simulink model "rocket_model"  (R2024a)
settings: Solver=VariableStepAuto  StartTime=0.0  StopTime=3  FixedStep=sample_time  RelTol=1e-3
undefined symbols (not defined in the file): armTVC, c_d, contact, fractalcoef, g, m, max_angle, sample_time
libraries: sharedtransform x4, sharedutil x3, slpidlib x2, aerolibutil x2, shared6dof x1, simulink x1, mspsensorlib x1, uavutilslib x1
settings Model: Creator=tommy  LastModifiedBy=tommy

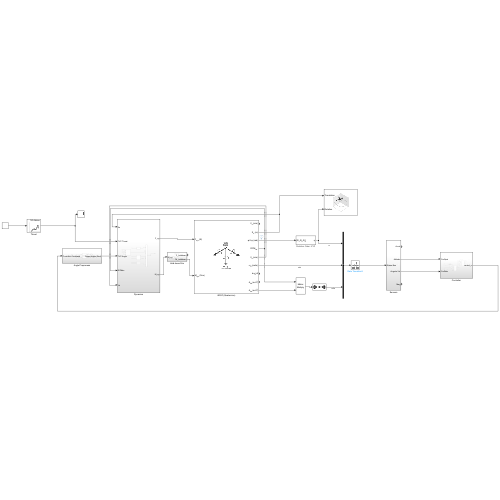
[thumbnail: Simulink's stored preview of the top-level diagram]
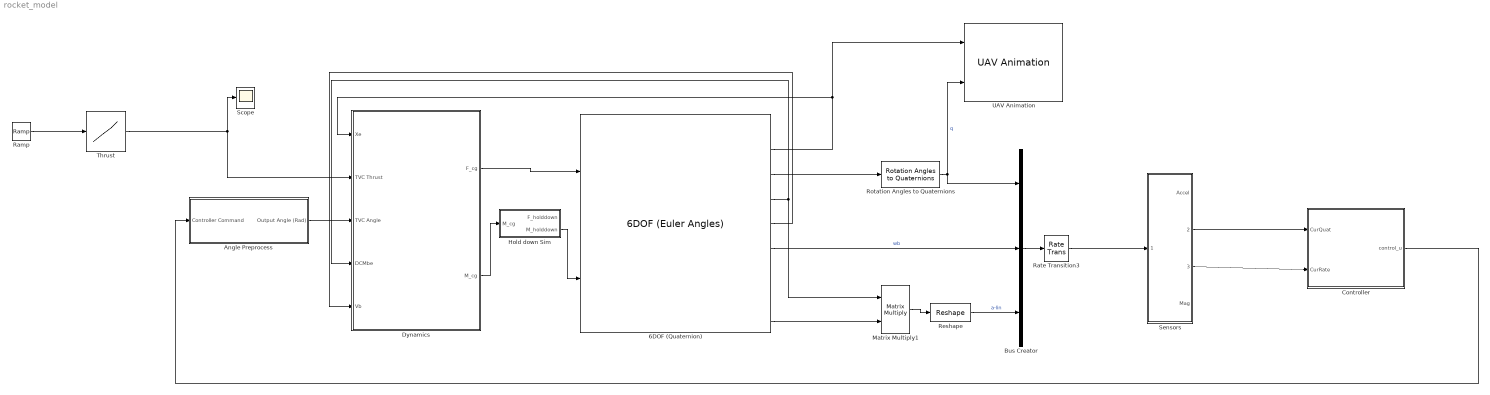
== system rocket_model ==
  6DOF (Quaternion) : shared6dof/6DOF (Euler Angles)  units=Metric (MKS)  mtype=Fixed  rep=Quaternion  xme_0=[0 0 0]  Vm_0=[0 0 0]  eul_0=[0, 0.2, 0]  pm_0=[0 0 0]  mass_0=m  mass_e=0.5  mass_f=2.0  inertia=inertia  inertia_e=eye(3)  inertia_f=2*eye(3)  k_quat=1  vre_flag=on  abi_flag=on  aMode=0  xme_statename=''  Vm_statename=''  eul_statename=''  quat_statename=''  pm_statename=''  mass_statename=''
      settings: LibrarySourceBlock=aerolib6dof2/6DOF (Quaternion)
  Angle Preprocess : Subsystem
  Bus Creator : BusCreator  Inputs=3
  Controller : Subsystem
  Dynamics : Subsystem
  Hold down Sim : Subsystem
  Matrix Multiply1 : Product  Multiplication=Matrix(*)
  Ramp : simulink/Sources/Ramp  slope=1  start=0  InitialOutput=0
  Rate Transition3 : RateTransition  OutPortSampleTime=sample_time
  Reshape : Reshape  OutputDimensionality=Row vector (2-D)
  Rotation Angles to Quaternions : sharedtransform/Rotation Angles to Quaternions  rotationOrder=XYZ  aMode=aMode
  Scope : Scope
  Sensors : Subsystem
  Thrust : Lookup_n-D  NumberOfTableDimensions=1  BreakpointsForDimension1=[0;0.15;0.186;0.206;0.242;0.252;0.277;0.333;0.359;0.374;0.394;0.435;0.476;0.521;0.643;0.725;0.821;0.898;1.025;1.142;1.259;1.396;1.569;1.757;1.895;2.027;2.042;2.052;2.063;2.09;4;10]  Table=[0;1.371;1.92;3.387;5.587;7.422;8.705;13.474;15.858;16.592;18.609;21.544;24.661;26.44;21.72;20.432;19.511;18.958;18.219;18.032;17.844;17.472;17.282;17.275;17.086;17.816;12.494;8.457;4.97;0;0;0]  InterpMethod=Akima spline  InternalRulePriority=Speed  RndMeth=Simplest
  UAV Animation : uavutilslib/UAV Animation  UAVType=Multirotor  UAVSize=1  InertialZDirection=Down  SampleTime=-1
  wires:
  Thrust/1 -> Dynamics/2(TVC Thrust), Scope/1
  6DOF (Quaternion)/4 -> Dynamics/4(DCMbe), Matrix Multiply1/1
  6DOF (Quaternion)/5 -> Dynamics/5(Vb)
  Ramp/1 -> Thrust/1
  6DOF (Quaternion)/2 -> UAV Animation/1, Dynamics/1(Xe)
  6DOF (Quaternion)/3 -> Rotation Angles to Quaternions/1
  Angle Preprocess/1(Output Angle (Rad)) -> Dynamics/3(TVC Angle)
  Controller/1(control_u) -> Angle Preprocess/1(Controller Command)
  Dynamics/2(M_cg) -> Hold down Sim/1(M_cg)
  Hold down Sim/2(M_holddown) -> 6DOF (Quaternion)/2
  6DOF (Quaternion)/9 -> Matrix Multiply1/2
  Matrix Multiply1/1 -> Reshape/1
  Dynamics/1(F_cg) -> 6DOF (Quaternion)/1
  Rotation Angles to Quaternions/1 -> Bus Creator/1, UAV Animation/2  "q"
  Reshape/1 -> Bus Creator/3  "a-lin"
  6DOF (Quaternion)/6 -> Bus Creator/2  "wb"
  Bus Creator/1 -> Rate Transition3/1
  Sensors/2(Attitude) -> Controller/1(CurQuat)
  Sensors/3(Angular Vel) -> Controller/2(CurRate)
  Rate Transition3/1 -> Sensors/1(States Bus)

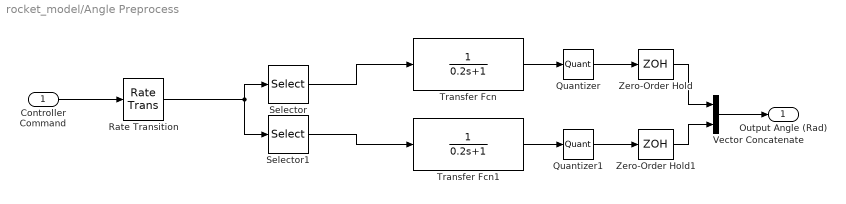
== system rocket_model/Angle Preprocess ==
  Controller Command : Inport
  Quantizer : Quantizer  QuantizationInterval=0.01745329251
  Quantizer1 : Quantizer  QuantizationInterval=0.01745329251
  Rate Transition : RateTransition  OutPortSampleTime=1/100
  Selector : Selector  InputPortWidth=3  IndexOptions=Index vector (dialog)  Indices=[1]  OutputSizes=1
  Selector1 : Selector  InputPortWidth=3  IndexOptions=Index vector (dialog)  Indices=[2]  OutputSizes=1
  Transfer Fcn : TransferFcn  Denominator=[0.2 1]
  Transfer Fcn1 : TransferFcn  Denominator=[0.2 1]
  Vector Concatenate : Concatenate
  Zero-Order Hold : ZeroOrderHold  SampleTime=1/100
  Zero-Order Hold1 : ZeroOrderHold  SampleTime=1/100
  Output Angle (Rad) : Outport
  wires:
  Vector Concatenate/1 -> Output Angle (Rad)/1
  Controller Command/1 -> Rate Transition/1
  Selector1/1 -> Transfer Fcn1/1
  Transfer Fcn/1 -> Quantizer/1
  Selector/1 -> Transfer Fcn/1
  Rate Transition/1 -> Selector1/1, Selector/1
  Quantizer/1 -> Zero-Order Hold/1
  Zero-Order Hold/1 -> Vector Concatenate/1
  Quantizer1/1 -> Zero-Order Hold1/1
  Zero-Order Hold1/1 -> Vector Concatenate/2
  Transfer Fcn1/1 -> Quantizer1/1

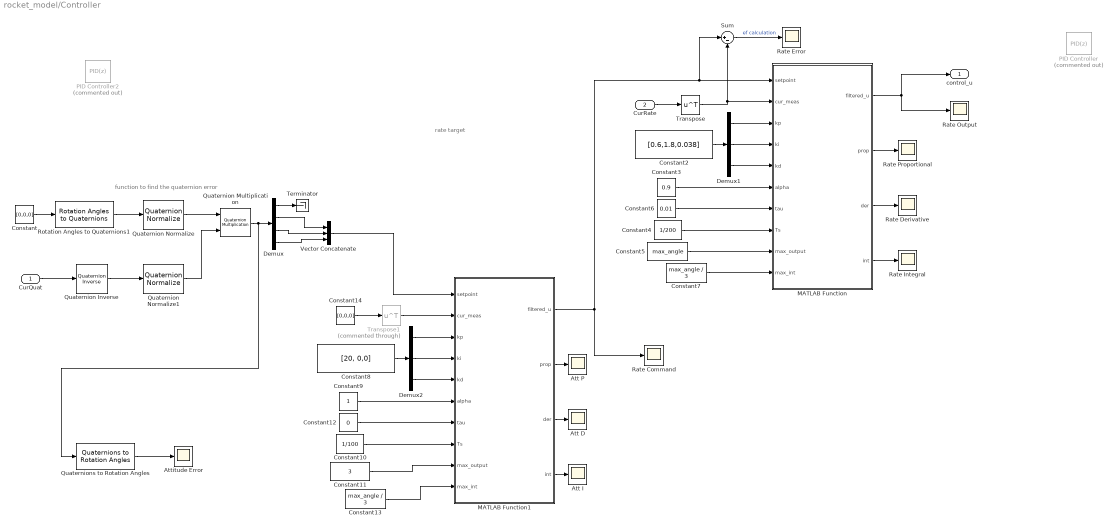
== system rocket_model/Controller ==
  note: rate target
  note: function to find the quaternion error
  CurQuat : Inport
  CurRate : Inport  Port=2
  Att D : Scope
  Att I : Scope
  Att P : Scope
  Attitude Error : Scope
  Constant : Constant  Value=[0,0,0]
  Constant10 : Constant  Value=1/100
  Constant11 : Constant  Value=3
  Constant12 : Constant  Value=0
  Constant13 : Constant  Value=max_angle / 3
  Constant14 : Constant  Value=[0,0,0]
  Constant2 : Constant  Value=[0.6,1.8,0.038]
  Constant3 : Constant  Value=0.9
  Constant4 : Constant  Value=1/200
  Constant5 : Constant  Value=max_angle
  Constant6 : Constant  Value=0.01
  Constant7 : Constant  Value=max_angle / 3
  Constant8 : Constant  Value=[20, 0,0]
  Constant9 : Constant
  Demux : Demux
  Demux1 : Demux  Outputs=3
  Demux2 : Demux  Outputs=3
  MATLAB Function : MATLAB Function  TreatAsAtomicUnit=on  SystemSampleTime=1/200
  MATLAB Function1 : MATLAB Function  TreatAsAtomicUnit=on  SystemSampleTime=1/200
  PID Controller : slpidlib/PID Controller  Commented=on  Controller=PID  Form=Parallel  TimeDomain=Discrete-time  UseExternalTs=off  SampleTime=sample_time  IntegratorMethod=Forward Euler  FilterMethod=Forward Euler  ControllerParametersSource=internal  P=6  I=20  UseKiTs=off  D=0.45  UseExternalDerivativeSource=off  N=30  UseFilter=on  TunerSelectOption=Transfer Function Based (PID Tuner App)  InitialConditionSource=internal  InitialConditionForIntegrator=0  InitialConditionForFilter=0  DifferentiatorICPrevScaledInput=0  ExternalReset=none  TrackingMode=off  Kt=1  LimitOutput=on  SatLimitsSource=internal  UpperSaturationLimit=0.1396  LowerSaturationLimit=-0.1396  LinearizeAsGain=on  AntiWindupMode=clamping  Kb=1/10  LimitIntegrator=off  UpperIntegratorSaturationLimit=inf  LowerIntegratorSaturationLimit=-inf  POutMin=[]  POutMax=[]  IOutMin=[]  IOutMax=[]  DOutMin=[]  DOutMax=[]  NOutMin=[]  NOutMax=[]  SumOutMin=[]  SumOutMax=[]  SaturationOutMin=[]  SaturationOutMax=[]  PParamMin=[]  PParamMax=[]  IParamMin=[]  IParamMax=[]  DParamMin=[]  DParamMax=[]  NParamMin=[]  NParamMax=[]  KbParamMin=[]  KbParamMax=[]  KtParamMin=[]  KtParamMax=[]  KbOutMin=[]  KbOutMax=[]  KtOutMin=[]  KtOutMax=[]  IntegratorOutMin=[]  IntegratorOutMax=[]  FilterOutMin=[]  FilterOutMax=[]  SumI1OutMin=[]  SumI1OutMax=[]  SumI2OutMin=[]  SumI2OutMax=[]  SumI3OutMin=[]  SumI3OutMax=[]  SumI4OutMin=[]  SumI4OutMax=[]  SumDOutMin=[]  SumDOutMax=[]  DifferentiatorOutMin=[]  DifferentiatorOutMax=[]  FilterDiffOutCoefMin=[]  FilterDiffOutCoefMax=[]  ReciprocalOutMin=[]  ReciprocalOutMax=[]  SumDenOutMin=[]  SumDenOutMax=[]  SumNumOutMin=[]  SumNumOutMax=[]  DivideOutMin=[]  DivideOutMax=[]  UdiffTsProdOutMin=[]  UdiffTsProdOutMax=[]  NTsProdOutMin=[]  NTsProdOutMax=[]  UintegralTsProdOutMin=[]  UintegralTsProdOutMax=[]  UngainTsProdOutMin=[]  UngainTsProdOutMax=[]  ClampingZeroOutDataTypeStr=Inherit: Inherit via back propagation  ClampingZeroOutMin=[]  ClampingZeroOutMax=[]  FilterDenConstantOutDataTypeStr=Inherit: Inherit via back propagation  FilterDenConstantOutMin=[]  FilterDenConstantOutMax=[]  PCopyOutDataTypeStr=Inherit: Inherit via back propagation  PCopyOutMin=[]  PCopyOutMax=[]  NCopyOutDataTypeStr=Inherit: Inherit via back propagation  NCopyOutMin=[]  NCopyOutMax=[]  IntegratorContinuousStateAttributes=''  IntegratorStateMustResolveToSignalObject=off  IntegratorRTWStateStorageClass=Auto  FilterContinuousStateAttributes=''  FilterStateMustResolveToSignalObject=off  FilterRTWStateStorageClass=Auto  ParallelPVariant=InternalParameters  IdealPVariant=Disabled  IVariant=InternalParameters  DVariant=InternalParameters  IntegratorVariant=Discrete  SatVariant=Enabled  AWVariant=DiscClampingParallel  PCopyVariant=Disabled  TRVariant=Disabled  FdbkBlocksVariant=Forward  IdealPFdbkVariant=Disabled  SatFdbkVariant=Disabled  DerivativeFilterVariant=ForwardEulerFilter  NVariant=InternalParameters  NCopyVariant=Disabled  FilterICVariant=InternalICsFilter  IntegratorICVariant=InternalICs  ExternalResetVariant=Disabled  TRSumVariant=Passthrough  SumFdbkVariant=Disabled  SumVariant=Sum_PID  TsampFilterVariant=InternalTs  TsampNgainVariant=Passthrough  TsampIntegralVariant=Disabled_SignalSpec  ExternalSaturationOutDataTypeStr=Inherit: Same as second input  DerivativeSourceVariant=ErrorSignal
  PID Controller2 : slpidlib/PID Controller  Commented=on  Controller=PID  Form=Parallel  TimeDomain=Discrete-time  UseExternalTs=off  SampleTime=sample_time  IntegratorMethod=Forward Euler  FilterMethod=Forward Euler  ControllerParametersSource=internal  P=30  I=0  UseKiTs=off  D=0.12  UseExternalDerivativeSource=off  N=1  UseFilter=on  TunerSelectOption=Transfer Function Based (PID Tuner App)  InitialConditionSource=internal  InitialConditionForIntegrator=0  InitialConditionForFilter=0  DifferentiatorICPrevScaledInput=0  ExternalReset=none  TrackingMode=off  Kt=1  LimitOutput=on  SatLimitsSource=internal  UpperSaturationLimit=1  LowerSaturationLimit=-1  LinearizeAsGain=on  AntiWindupMode=clamping  Kb=1  LimitIntegrator=off  UpperIntegratorSaturationLimit=inf  LowerIntegratorSaturationLimit=-inf  POutMin=[]  POutMax=[]  IOutMin=[]  IOutMax=[]  DOutMin=[]  DOutMax=[]  NOutMin=[]  NOutMax=[]  SumOutMin=[]  SumOutMax=[]  SaturationOutMin=[]  SaturationOutMax=[]  PParamMin=[]  PParamMax=[]  IParamMin=[]  IParamMax=[]  DParamMin=[]  DParamMax=[]  NParamMin=[]  NParamMax=[]  KbParamMin=[]  KbParamMax=[]  KtParamMin=[]  KtParamMax=[]  KbOutMin=[]  KbOutMax=[]  KtOutMin=[]  KtOutMax=[]  IntegratorOutMin=[]  IntegratorOutMax=[]  FilterOutMin=[]  FilterOutMax=[]  SumI1OutMin=[]  SumI1OutMax=[]  SumI2OutMin=[]  SumI2OutMax=[]  SumI3OutMin=[]  SumI3OutMax=[]  SumI4OutMin=[]  SumI4OutMax=[]  SumDOutMin=[]  SumDOutMax=[]  DifferentiatorOutMin=[]  DifferentiatorOutMax=[]  FilterDiffOutCoefMin=[]  FilterDiffOutCoefMax=[]  ReciprocalOutMin=[]  ReciprocalOutMax=[]  SumDenOutMin=[]  SumDenOutMax=[]  SumNumOutMin=[]  SumNumOutMax=[]  DivideOutMin=[]  DivideOutMax=[]  UdiffTsProdOutMin=[]  UdiffTsProdOutMax=[]  NTsProdOutMin=[]  NTsProdOutMax=[]  UintegralTsProdOutMin=[]  UintegralTsProdOutMax=[]  UngainTsProdOutMin=[]  UngainTsProdOutMax=[]  ClampingZeroOutDataTypeStr=Inherit: Inherit via back propagation  ClampingZeroOutMin=[]  ClampingZeroOutMax=[]  FilterDenConstantOutDataTypeStr=Inherit: Inherit via back propagation  FilterDenConstantOutMin=[]  FilterDenConstantOutMax=[]  PCopyOutDataTypeStr=Inherit: Inherit via back propagation  PCopyOutMin=[]  PCopyOutMax=[]  NCopyOutDataTypeStr=Inherit: Inherit via back propagation  NCopyOutMin=[]  NCopyOutMax=[]  IntegratorContinuousStateAttributes=''  IntegratorStateMustResolveToSignalObject=off  IntegratorRTWStateStorageClass=Auto  FilterContinuousStateAttributes=''  FilterStateMustResolveToSignalObject=off  FilterRTWStateStorageClass=Auto  ParallelPVariant=InternalParameters  IdealPVariant=Disabled  IVariant=InternalParameters  DVariant=InternalParameters  IntegratorVariant=Discrete  SatVariant=Enabled  AWVariant=DiscClampingParallel  PCopyVariant=Disabled  TRVariant=Disabled  FdbkBlocksVariant=Forward  IdealPFdbkVariant=Disabled  SatFdbkVariant=Disabled  DerivativeFilterVariant=ForwardEulerFilter  NVariant=InternalParameters  NCopyVariant=Disabled  FilterICVariant=InternalICsFilter  IntegratorICVariant=InternalICs  ExternalResetVariant=Disabled  TRSumVariant=Passthrough  SumFdbkVariant=Disabled  SumVariant=Sum_PID  TsampFilterVariant=InternalTs  TsampNgainVariant=Passthrough  TsampIntegralVariant=Disabled_SignalSpec  ExternalSaturationOutDataTypeStr=Inherit: Same as second input  DerivativeSourceVariant=ErrorSignal
  Quaternion Inverse : aerolibutil/Quaternion Inverse
  Quaternion Multiplication : aerolibutil/Quaternion Multiplication
  Quaternion Normalize : sharedutil/Quaternion Normalize  aMode=aMode
  Quaternion Normalize1 : sharedutil/Quaternion Normalize  aMode=aMode
  Quaternions to Rotation Angles : sharedtransform/Quaternions to Rotation Angles  rotationOrder=XYZ  aMode=aMode
  Rate Command : Scope
  Rate Derivative : Scope
  Rate Error : Scope
  Rate Integral : Scope
  Rate Output : Scope
  Rate Proportional : Scope
  Rotation Angles to Quaternions1 : sharedtransform/Rotation Angles to Quaternions  rotationOrder=XYZ  aMode=aMode
  Sum : Sum  Inputs=|+-
  Terminator : Terminator
  Transpose : Math  Operator=transpose
  Transpose1 : Math  Commented=through  Operator=transpose
  Vector Concatenate : Concatenate  NumInputs=3
  control_u : Outport
  wires:
  Constant/1 -> Rotation Angles to Quaternions1/1
  CurQuat/1 -> Quaternion Inverse/1
  Rotation Angles to Quaternions1/1 -> Quaternion Normalize/1
  Quaternion Inverse/1 -> Quaternion Normalize1/1
  Quaternion Normalize/1 -> Quaternion Multiplication/1
  Quaternion Normalize1/1 -> Quaternion Multiplication/2
  Demux/1 -> Terminator/1
  Quaternion Multiplication/1 -> Quaternions to Rotation Angles/1, Demux/1
  Demux/2 -> Vector Concatenate/1
  Demux/3 -> Vector Concatenate/2
  Demux/4 -> Vector Concatenate/3
  Quaternions to Rotation Angles/1 -> Attitude Error/1
  MATLAB Function/1(filtered_u) -> control_u/1, Rate Output/1
  Vector Concatenate/1 -> MATLAB Function1/1(setpoint)
  CurRate/1 -> Transpose/1
  Sum/1 -> Rate Error/1  "ef calculation"
  MATLAB Function1/1(filtered_u) -> Sum/1, MATLAB Function/1(setpoint), Rate Command/1
  Constant2/1 -> Demux1/1
  Demux1/1 -> MATLAB Function/3(kp)
  Demux1/2 -> MATLAB Function/4(ki)
  Demux1/3 -> MATLAB Function/5(kd)
  Constant3/1 -> MATLAB Function/6(alpha)
  Constant4/1 -> MATLAB Function/8(Ts)
  Constant5/1 -> MATLAB Function/9(max_output)
  Transpose/1 -> Sum/2, MATLAB Function/2(cur_meas)
  Constant6/1 -> MATLAB Function/7(tau)
  MATLAB Function/4(int) -> Rate Integral/1
  MATLAB Function/3(der) -> Rate Derivative/1
  MATLAB Function/2(prop) -> Rate Proportional/1
  Constant7/1 -> MATLAB Function/10(max_int)
  Constant12/1 -> MATLAB Function1/7(tau)
  Constant13/1 -> MATLAB Function1/10(max_int)
  Constant9/1 -> MATLAB Function1/6(alpha)
  Constant10/1 -> MATLAB Function1/8(Ts)
  Demux2/1 -> MATLAB Function1/3(kp)
  Constant11/1 -> MATLAB Function1/9(max_output)
  Constant8/1 -> Demux2/1
  Demux2/2 -> MATLAB Function1/4(ki)
  Demux2/3 -> MATLAB Function1/5(kd)
  Constant14/1 -> Transpose1/1
  Transpose1/1 -> MATLAB Function1/2(cur_meas)
  MATLAB Function1/2(prop) -> Att P/1
  MATLAB Function1/3(der) -> Att D/1
  MATLAB Function1/4(int) -> Att I/1

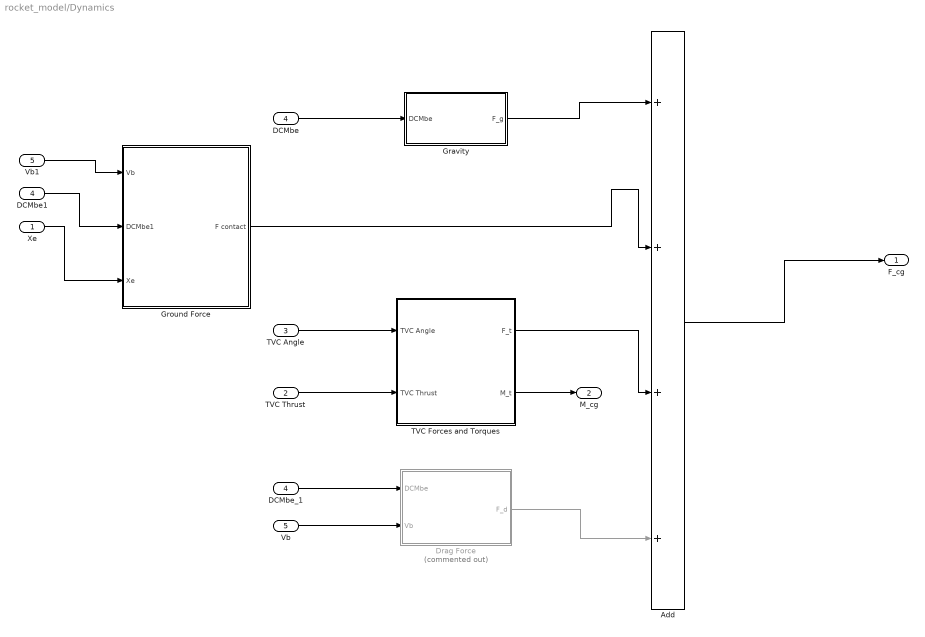
== system rocket_model/Dynamics ==
  Xe : Inport
  TVC Thrust : Inport  Port=2
  TVC Angle : Inport  Port=3
  DCMbe : Inport  Port=4
  Vb : Inport  Port=5
  Add : Sum  Inputs=++++
  DCMbe1 : InportShadow  Port=4
  DCMbe_1 : InportShadow  Port=4
  Drag Force : Subsystem  Commented=on
  Gravity : Subsystem
  Ground Force : Subsystem
  TVC Forces and Torques : Subsystem
  Vb1 : InportShadow  Port=5
  F_cg : Outport
  M_cg : Outport  Port=2
  wires:
  Add/1 -> F_cg/1
  DCMbe_1/1 -> Drag Force/1(DCMbe)
  TVC Forces and Torques/1(F_t) -> Add/3
  Vb/1 -> Drag Force/2(Vb)
  Gravity/1(F_g) -> Add/1
  TVC Thrust/1 -> TVC Forces and Torques/2(TVC Thrust)
  TVC Forces and Torques/2(M_t) -> M_cg/1
  DCMbe/1 -> Gravity/1(DCMbe)
  TVC Angle/1 -> TVC Forces and Torques/1(TVC Angle)
  Drag Force/1(F_d) -> Add/4
  DCMbe1/1 -> Ground Force/2(DCMbe1)
  Xe/1 -> Ground Force/3(Xe)
  Ground Force/1(F contact) -> Add/2
  Vb1/1 -> Ground Force/1(Vb)

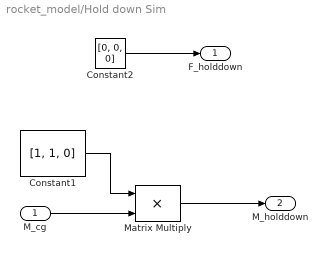
== system rocket_model/Hold down Sim ==
  M_cg : Inport
  Constant1 : Constant  Value=[1, 1, 0]
  Constant2 : Constant  Value=[0, 0, 0]
  Matrix Multiply : Product
  F_holddown : Outport
  M_holddown : Outport  Port=2
  wires:
  Constant1/1 -> Matrix Multiply/1
  Matrix Multiply/1 -> M_holddown/1
  M_cg/1 -> Matrix Multiply/2
  Constant2/1 -> F_holddown/1

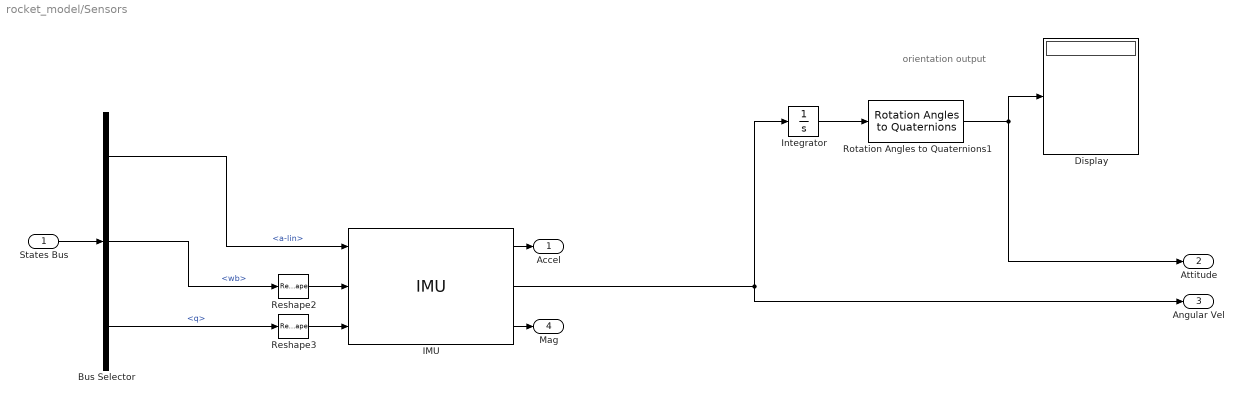
== system rocket_model/Sensors ==
  note: orientation output
  States Bus : Inport
  Bus Selector : BusSelector  OutputSignals=a-lin,wb,q
  Display : Display
  IMU : mspsensorlib/IMU  DispRefFrame=NED  TemperaturePort=off  Temperature=0  MagneticFieldPort=off  MagneticFieldNED=[ 27.5550, -2.4169, -16.0849 ]  MagneticFieldENU=[ -2.4169, 27.5550, 16.0849 ]  SeedDouble=67  SimulateUsing=Interpreted execution  AccelParamsMeasurementRange=Inf  AccelParamsResolution=0  AccelParamsConstantBias=[ 0, 0, 0 ]  AccelParamsAxesMisalignment=[ 100, 0, 0; 0, 100, 0; 0, 0, 100 ]  AccelParamsNoiseDensity=[ 0, 0, 0 ]  AccelParamsBiasInstability=[ 0, 0, 0 ]  AccelParamsBiasInstabilityNumerator=fractalcoef().Numerator  AccelParamsBiasInstabilityDenominator=fractalcoef().Denominator  AccelParamsRandomWalk=[ 0, 0, 0 ]  AccelParamsNoiseType=double-sided  AccelParamsTemperatureBias=[ 0, 0, 0 ]  AccelParamsTemperatureScaleFactor=[ 0, 0, 0 ]  GyroParamsMeasurementRange=Inf  GyroParamsResolution=0  GyroParamsConstantBias=[ 0, 0, 0 ]  GyroParamsAxesMisalignment=[ 100, 0, 0; 0, 100, 0; 0, 0, 100 ]  GyroParamsAccelerationBias=[ 0, 0, 0 ]  GyroParamsNoiseDensity=[ 0.0000663, 0.0000663, 0.00006635]  GyroParamsBiasInstability=[ 0, 0, 0 ]  GyroParamsBiasInstabilityNumerator=fractalcoef().Numerator  GyroParamsBiasInstabilityDenominator=fractalcoef().Denominator  GyroParamsRandomWalk=[ 0, 0, 0 ]  GyroParamsNoiseType=double-sided  GyroParamsTemperatureBias=[ 0, 0, 0 ]  GyroParamsTemperatureScaleFactor=[ 0, 0, 0 ]  MagParamsMeasurementRange=Inf  MagParamsResolution=0  MagParamsConstantBias=[ 0, 0, 0 ]  MagParamsAxesMisalignment=[ 100, 0, 0; 0, 100, 0; 0, 0, 100 ]  MagParamsNoiseDensity=[ 0, 0, 0 ]  MagParamsBiasInstability=[ 0, 0, 0 ]  MagParamsBiasInstabilityNumerator=fractalcoef().Numerator  MagParamsBiasInstabilityDenominator=fractalcoef().Denominator  MagParamsRandomWalk=[ 0, 0, 0 ]  MagParamsNoiseType=double-sided  MagParamsTemperatureBias=[ 0, 0, 0 ]  MagParamsTemperatureScaleFactor=[ 0, 0, 0 ]
  Integrator : Integrator  InitialCondition=[0, 0.2, 0]
  Reshape2 : Reshape  OutputDimensionality=Row vector (2-D)
  Reshape3 : Reshape  OutputDimensionality=Row vector (2-D)
  Rotation Angles to Quaternions1 : sharedtransform/Rotation Angles to Quaternions  rotationOrder=XYZ  aMode=aMode
  Accel : Outport
  Attitude : Outport  Port=2
  Angular Vel : Outport  Port=3
  Mag : Outport  Port=4
  wires:
  Integrator/1 -> Rotation Angles to Quaternions1/1
  IMU/1 -> Accel/1
  Rotation Angles to Quaternions1/1 -> Attitude/1, Display/1
  IMU/3 -> Mag/1
  IMU/2 -> Angular Vel/1, Integrator/1
  Reshape3/1 -> IMU/3
  Reshape2/1 -> IMU/2
  States Bus/1 -> Bus Selector/1
  Bus Selector/1 -> IMU/1  "<a-lin>"
  Bus Selector/3 -> Reshape3/1  "<q>"
  Bus Selector/2 -> Reshape2/1  "<wb>"

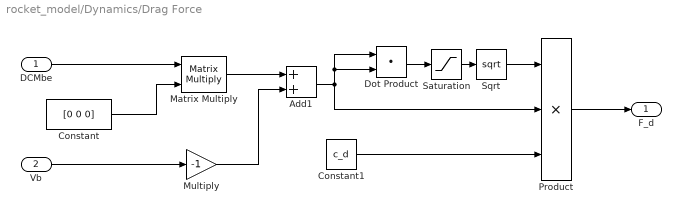
== system rocket_model/Dynamics/Drag Force ==
  DCMbe : Inport
  Vb : Inport  Port=2
  Add1 : Sum
  Constant : Constant  Value=[0 0 0]
  Constant1 : Constant  Value=c_d
  Dot Product : DotProduct  OutDataTypeStr=Inherit: Inherit via internal rule
  Matrix Multiply : Product  Multiplication=Matrix(*)
  Multiply : Gain  Gain=-1
  Product : Product  Inputs=3
  Saturation : Saturate  UpperLimit=inf  LowerLimit=0.00001
  Sqrt : Sqrt
  F_d : Outport
  wires:
  Dot Product/1 -> Saturation/1
  Multiply/1 -> Add1/2
  Constant/1 -> Matrix Multiply/2
  Matrix Multiply/1 -> Add1/1
  Add1/1 -> Product/2, Dot Product/1, Dot Product/2
  Vb/1 -> Multiply/1
  DCMbe/1 -> Matrix Multiply/1
  Sqrt/1 -> Product/1
  Saturation/1 -> Sqrt/1
  Product/1 -> F_d/1
  Constant1/1 -> Product/3

== system rocket_model/Dynamics/Gravity ==
  DCMbe : Inport
  Constant : Constant  Value=[0 0 g]
  Matrix Multiply : Product  Multiplication=Matrix(*)
  Multiply : Gain  Gain=m
  F_g : Outport
  wires:
  Multiply/1 -> Matrix Multiply/2
  DCMbe/1 -> Matrix Multiply/1
  Constant/1 -> Multiply/1
  Matrix Multiply/1 -> F_g/1

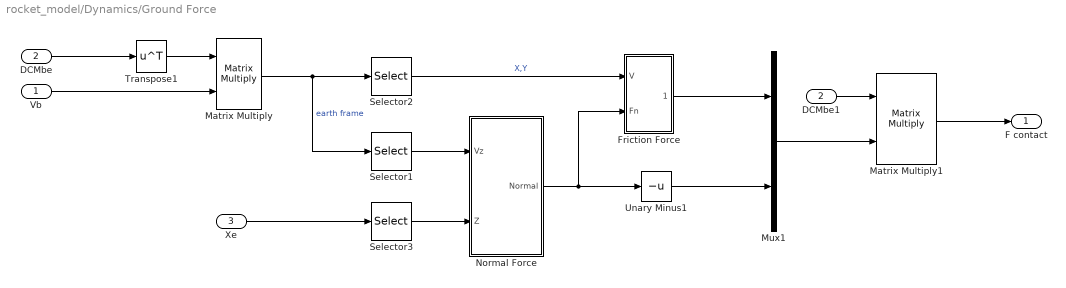
== system rocket_model/Dynamics/Ground Force ==
  Vb : Inport
  DCMbe1 : Inport  Port=2
  Xe : Inport  Port=3
  DCMbe : InportShadow  Port=2
  Friction Force : Subsystem
  Matrix Multiply : Product  Multiplication=Matrix(*)
  Matrix Multiply1 : Product  Multiplication=Matrix(*)
  Mux1 : Mux  Inputs=2
  Normal Force : Subsystem
  Selector1 : Selector  InputPortWidth=3  IndexOptions=Index vector (dialog)  Indices=[3]  OutputSizes=1
  Selector2 : Selector  InputPortWidth=3  IndexOptions=Index vector (dialog)  Indices=[1,2]  OutputSizes=1
  Selector3 : Selector  InputPortWidth=3  IndexOptions=Index vector (dialog)  Indices=[3]  OutputSizes=1
  Transpose1 : Math  Operator=transpose
  Unary Minus1 : UnaryMinus
  F contact : Outport
  wires:
  Matrix Multiply1/1 -> F contact/1
  Friction Force/1(Friction) -> Mux1/1
  Xe/1 -> Selector3/1
  Vb/1 -> Matrix Multiply/2
  Selector3/1 -> Normal Force/2(Z)
  Matrix Multiply/1 -> Selector1/1, Selector2/1  "earth frame"
  Mux1/1 -> Matrix Multiply1/2
  Selector2/1 -> Friction Force/1(V)  "X,Y"
  Selector1/1 -> Normal Force/1(Vz)
  DCMbe1/1 -> Matrix Multiply1/1
  DCMbe/1 -> Transpose1/1
  Transpose1/1 -> Matrix Multiply/1
  Unary Minus1/1 -> Mux1/2
  Normal Force/1(Normal) -> Unary Minus1/1, Friction Force/2(Fn)

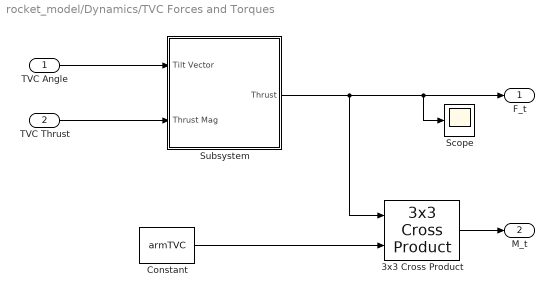
== system rocket_model/Dynamics/TVC Forces and Torques ==
  TVC Angle : Inport
  TVC Thrust : Inport  Port=2
  3x3 Cross Product : sharedutil/3x3 Cross Product  aMode=aMode
      settings: LibrarySourceBlock=aerolibutil/3x3 Cross Product
  Constant : Constant  Value=armTVC
  Scope : Scope
  Subsystem : Subsystem
  F_t : Outport
  M_t : Outport  Port=2
  wires:
  TVC Angle/1 -> Subsystem/1(Tilt Vector)
  TVC Thrust/1 -> Subsystem/2(Thrust Mag)
  Subsystem/1(Thrust) -> 3x3 Cross Product/1, Scope/1, F_t/1
  Constant/1 -> 3x3 Cross Product/2
  3x3 Cross Product/1 -> M_t/1

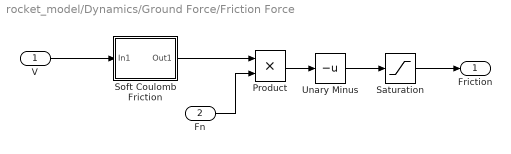
== system rocket_model/Dynamics/Ground Force/Friction Force ==
  V : Inport
  Fn : Inport  Port=2
  Product : Product
  Saturation : Saturate  UpperLimit=contact.translation.maxFriction  LowerLimit=-contact.translation.maxFriction
  Soft Coulomb Friction : Subsystem
  Unary Minus : UnaryMinus
  Friction : Outport
  wires:
  Fn/1 -> Product/2
  Soft Coulomb Friction/1(Out1) -> Product/1
  Product/1 -> Unary Minus/1
  V/1 -> Soft Coulomb Friction/1(In1)
  Unary Minus/1 -> Saturation/1
  Saturation/1 -> Friction/1

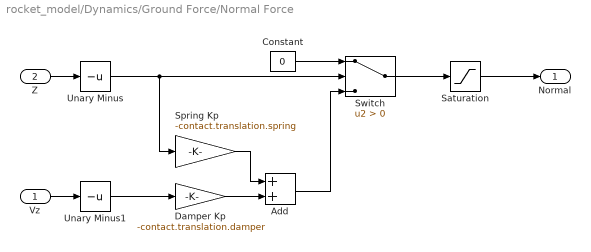
== system rocket_model/Dynamics/Ground Force/Normal Force ==
  Vz : Inport
  Z : Inport  Port=2
  Add : Sum
  Constant : Constant  Value=0
  Damper Kp : Gain  Gain=-contact.translation.damper
  Saturation : Saturate  UpperLimit=contact.translation.maxNormal  LowerLimit=0
  Spring Kp : Gain  Gain=-contact.translation.spring
  Switch : Switch  Criteria=u2 > Threshold  SaturateOnIntegerOverflow=off  InputSameDT=off
  Unary Minus : UnaryMinus
  Unary Minus1 : UnaryMinus
  Normal : Outport
  wires:
  Constant/1 -> Switch/1
  Z/1 -> Unary Minus/1
  Switch/1 -> Saturation/1
  Damper Kp/1 -> Add/2
  Add/1 -> Switch/3
  Spring Kp/1 -> Add/1
  Vz/1 -> Unary Minus1/1
  Saturation/1 -> Normal/1
  Unary Minus/1 -> Spring Kp/1, Switch/2
  Unary Minus1/1 -> Damper Kp/1

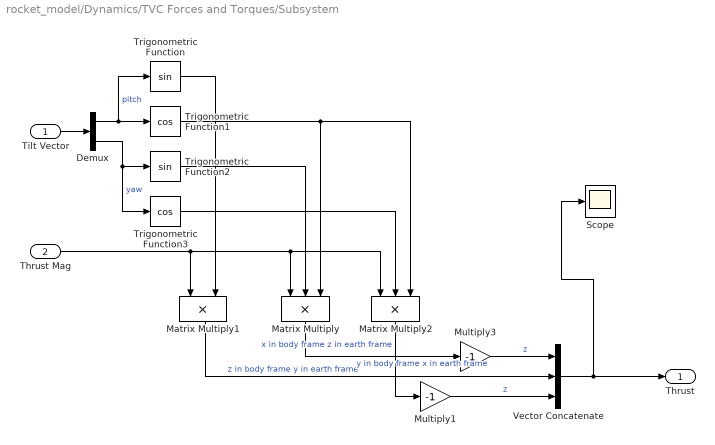
== system rocket_model/Dynamics/TVC Forces and Torques/Subsystem ==
  Tilt Vector : Inport
  Thrust Mag : Inport  Port=2
  Demux : Demux  Outputs=2
  Matrix Multiply : Product  Inputs=3
  Matrix Multiply1 : Product
  Matrix Multiply2 : Product  Inputs=3
  Multiply1 : Gain  Gain=-1
  Multiply3 : Gain  Gain=-1
  Scope : Scope
  Trigonometric Function : Trigonometry
  Trigonometric Function1 : Trigonometry  Operator=cos
  Trigonometric Function2 : Trigonometry
  Trigonometric Function3 : Trigonometry  Operator=cos
  Vector Concatenate : Concatenate  NumInputs=3
  Thrust : Outport
  wires:
  Trigonometric Function2/1 -> Matrix Multiply/2
  Demux/2 -> Trigonometric Function3/1, Trigonometric Function2/1  "yaw"
  Matrix Multiply1/1 -> Vector Concatenate/2  "z in body frame y in earth frame"
  Tilt Vector/1 -> Demux/1
  Trigonometric Function1/1 -> Matrix Multiply/3, Matrix Multiply2/3
  Demux/1 -> Trigonometric Function/1, Trigonometric Function1/1  "pitch"
  Trigonometric Function3/1 -> Matrix Multiply2/2
  Thrust Mag/1 -> Matrix Multiply2/1, Matrix Multiply/1, Matrix Multiply1/1
  Vector Concatenate/1 -> Scope/1, Thrust/1
  Trigonometric Function/1 -> Matrix Multiply1/2
  Matrix Multiply2/1 -> Multiply1/1  "x in body frame z in earth frame"
  Multiply1/1 -> Vector Concatenate/3  "z"
  Multiply3/1 -> Vector Concatenate/1  "z"
  Matrix Multiply/1 -> Multiply3/1  "y in body frame x in earth frame"

== system rocket_model/Dynamics/Ground Force/Friction Force/Soft Coulomb Friction ==
  note: Pennestrì, E., Rossi, V., Salvini, P. et al. Review and comparison of dry friction force models. Nonlinear Dyn 83, 1785–1801 (2016). https://doi.org/10.1007/s11071-015-2485-3
  In1 : Inport
  Tanh : Trigonometry  Operator=tanh
  friction coefficient : Gain  Gain=contact.translation.friction
  vd : Gain  Gain=1/contact.translation.vd
  Out1 : Outport
  wires:
  In1/1 -> vd/1
  vd/1 -> Tanh/1
  Tanh/1 -> friction coefficient/1
  friction coefficient/1 -> Out1/1

== matlab function rocket_model/Controller/MATLAB Function1 ==
  data: setpoint input; filtered_u output; prop output; der output; cur_meas input; kp input; ki input; kd input; alpha input; tau input; Ts input; max_output input; int output; max_int input
function [filtered_u, prop, der, int]   = PID_Simulink(setpoint, cur_meas, kp, ki, kd, alpha, tau, Ts, max_output, max_int)
% PID_Simulink: A basic PID controller function for Simulink with support for 3D vector inputs.
% Inputs:
%   reference  - Desired setpoint (3x1 vector)
%   meas_y     - Measured output (3x1 vector)
%   kp, ki, kd - PID gains (scalars)
%   alpha      - Filter coefficient (scalar)
%   Ts         - Sampling time (scalar)
%   max_output - Maximum output value (scalar)
% Outputs:
%   control_u  - PID control signal (3x1 vector)

% Declare persistent variables for integral and filtered error states
persistent integral_att old_ef_att old_uf_att

% Initialize persistent variables at the first execution
if isempty(integral_att)
    integral_att = zeros(3, 1); % Initialize as zero for a 3D vector
end
if isempty(old_ef_att)
    old_ef_att = zeros(3, 1); % Initialize as zero for a 3D vector
end
if isempty(old_uf_att)
    old_uf_att = zeros(3, 1);
end

% Calculate the error
error = setpoint - cur_meas;

% Filtered error
ef = alpha .* error + (1 - alpha) .* old_ef_att;

% Derivative of the filtered error
derivative = (ef - old_ef_att) ./ Ts;

% PID formula
control_u = kp .* error + ki .* integral_att + kd .* derivative;

% Clamp the output for each dimension
for i = 1:3
    if control_u(i) > max_output
        control_u(i) = max_output;
    elseif control_u(i) < -max_output
        control_u(i) = -max_output;
    elseif abs(integral_att(i)) < max_int
        integral_att(i) = integral_att(i) + error(i) * Ts;
    end
end

alpha_lpf = Ts / (Ts + tau);
filtered_u = alpha_lpf .* control_u + (1 - alpha_lpf) .* old_uf_att;


% Update persistent variables for the next iteration
old_ef_att = ef;
old_uf_att = filtered_u;
int = integral_att;
prop = kp .* error;
der = derivative;

end

== matlab function rocket_model/Controller/MATLAB Function ==
  data: setpoint input; filtered_u output; prop output; der output; cur_meas input; kp input; ki input; kd input; alpha input; tau input; Ts input; max_output input; int output; max_int input
function [filtered_u, prop, der, int]   = PID_Simulink(setpoint, cur_meas, kp, ki, kd, alpha, tau, Ts, max_output, max_int)
% PID_Simulink: A basic PID controller function for Simulink with support for 3D vector inputs.
% Inputs:
%   reference  - Desired setpoint (3x1 vector)
%   meas_y     - Measured output (3x1 vector)
%   kp, ki, kd - PID gains (scalars)
%   alpha      - Filter coefficient (scalar)
%   Ts         - Sampling time (scalar)
%   max_output - Maximum output value (scalar)
% Outputs:
%   control_u  - PID control signal (3x1 vector)

% Declare persistent variables for integral and filtered error states
persistent integral old_ef old_uf

% Initialize persistent variables at the first execution
if isempty(integral)
    integral = zeros(3, 1); % Initialize as zero for a 3D vector
end
if isempty(old_ef)
    old_ef = zeros(3, 1); % Initialize as zero for a 3D vector
end
if isempty(old_uf)
    old_uf = zeros(3, 1);
end

% Calculate the error
error = setpoint - cur_meas;

% Filtered error
ef = alpha .* error + (1 - alpha) .* old_ef;

% Derivative of the filtered error
derivative = (ef - old_ef) ./ Ts;

% PID formula
control_u = kp .* error + ki .* integral + kd .* derivative;

% Clamp the output for each dimension
for i = 1:3
    if control_u(i) > max_output
        control_u(i) = max_output;
    elseif control_u(i) < -max_output
        control_u(i) = -max_output;
    elseif abs(integral(i)) < max_int
        integral(i) = integral(i) + error(i) * Ts;
    end
end

alpha_lpf = Ts / (Ts + tau);
filtered_u = alpha_lpf .* control_u + (1 - alpha_lpf) .* old_uf;


% Update persistent variables for the next iteration
old_ef = ef;
old_uf = filtered_u;
int = integral;
prop = kp .* error;
der = derivative;

end
